simulink subsystem "RigidRod"  (R2022b)
settings: Solver=VariableStepAuto  StartTime=0.0  StopTime=10.0  RelTol=1e-3
libraries: simulink x1
settings Model: Creator=lukasz  LastModifiedBy=lukasz

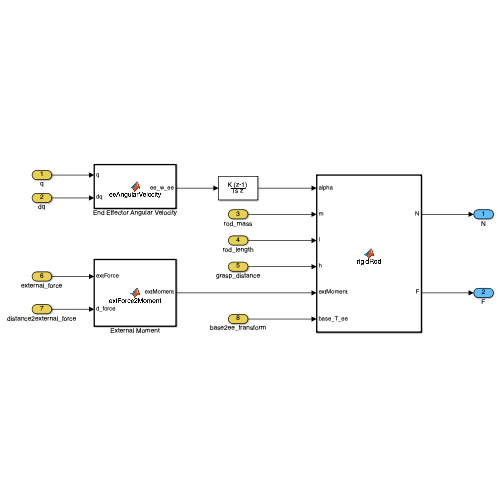
[thumbnail: Simulink's stored preview of the top-level diagram]
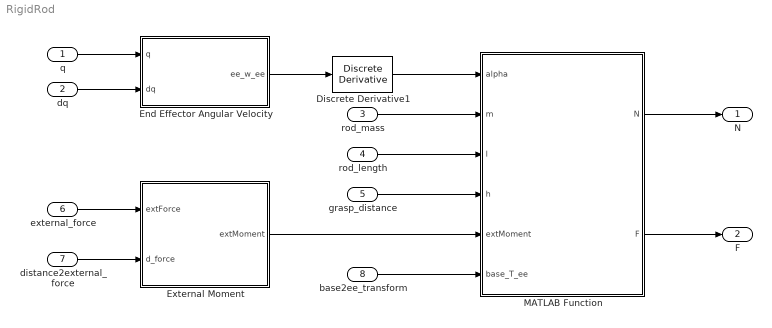
== system RigidRod ==
  q : Inport
  dq : Inport  Port=2
  rod_mass : Inport  Port=3
  rod_length : Inport  Port=4
  grasp_distance : Inport  Port=5
  external_force : Inport  Port=6
  distance2external_force : Inport  Port=7
  base2ee_transform : Inport  Port=8
  Discrete Derivative1 : simulink/Discrete/Discrete Derivative  gainval=1.0  ICPrevScaledInput="[ 0 ; 0;  0]"  OutMin=[]  OutMax=[]  OutDataType=fixdt(1, 16)  OutScaling=2^-10  DoSatur=off
  End Effector Angular Velocity : MATLAB Function  TreatAsAtomicUnit=on
  External Moment : MATLAB Function  TreatAsAtomicUnit=on
  MATLAB Function : MATLAB Function  TreatAsAtomicUnit=on
  N : Outport
  F : Outport  Port=2
  wires:
  dq/1 -> End Effector Angular Velocity/2(dq)
  q/1 -> End Effector Angular Velocity/1(q)
  MATLAB Function/1(N) -> N/1
  End Effector Angular Velocity/1(ee_w_ee) -> Discrete Derivative1/1
  rod_mass/1 -> MATLAB Function/2(m)
  rod_length/1 -> MATLAB Function/3(l)
  grasp_distance/1 -> MATLAB Function/4(h)
  MATLAB Function/2(F) -> F/1
  distance2external_force/1 -> External Moment/2(d_force)
  base2ee_transform/1 -> MATLAB Function/6(base_T_ee)
  Discrete Derivative1/1 -> MATLAB Function/1(alpha)
  External Moment/1(extMoment) -> MATLAB Function/5(extMoment)
  external_force/1 -> External Moment/1(extForce)

== matlab function RigidRod/End Effector Angular Velocity ==
  data: q input; ee_w_ee output; dq input
function ee_w_ee = eeAngularVelocity(q, dq)

q1 = q(1);
q2 = q(2);
q3 = q(3);

dq1 = dq(1);
dq2 = dq(2);
dq3 = dq(3);

w1 = 0;
w2 = cos(q3)*(-sin(q1)*cos(q2)*dq1 + sin(q2)*(cos(q1)*dq1 + dq2)) - ...
    sin(q3)*(sin(q1)*sin(q2)*dq1 + cos(q2)*(cos(q1)*dq1 + dq2) + dq3);
w3 = sin(q3)*(-sin(q1)*cos(q2)*dq1 + sin(q2)*(cos(q1)*dq1 + dq2)) + ...
    cos(q3)*(sin(q1)*sin(q2)*dq1 + cos(q2)*(cos(q1)*dq1 + dq2) + dq3);

ee_w_ee = [w1; w2; w3];

== matlab function RigidRod/MATLAB Function ==
  data: alpha input; N output; m input; l input; h input; F output; extMoment input; base_T_ee input
function [N, F] = rigidRod(alpha, m, l, h, extMoment, base_T_ee)

G = ee_T_base(1:3,1:3)*[0;0;9.81]; % rotate gravity vector into ee frame
I = (1/3)* m * (l^3 - 3*l*h + 3*h^2); % inertia of rod at grasp location
% moment of inertia + moment from gravity + any externally applied force
% moment
N = I*alpha + m*G*(l/2 - h) + extMoment; 
% gravitational force acting at grasp location
F = m*G;

== matlab function RigidRod/External Moment ==
  data: extForce input; extMoment output; d_force input
function extMoment = extForce2Moment(extForce, d_force)

extMoment = extForce*d_force;
